simulink model "AUAV_V3_TestMavLink"  (Simulink 7.8)
settings: Solver=FixedStepDiscrete  StartTime=0.0  StopTime=10.0  FixedStep=T  RelTol=1e-3
PreLoadFcn:
  | T = 0.005;
  | MavlinkBus;
values from neighbouring files (symbols this model uses):
  mavlink_raw_imu_t = Simulink.Bus    [MavlinkBus.m]
undefined symbols (not defined in the file or in its folder): A0, A2, A3, A6, B0, D0, F2, F3, G15, P127, P16, P64, P82, P83, P98, P99, Pin, Timer
libraries: MCHP_Blockset x22, simulink x4
Description:
  | Rapid Prototyping model.
  | Require the MPLAB Blockset for Simulink v3.30 or above. [http://www.microchip.com/SimulinkBlocks]
  | Author: Lubin Kerhuel
  | 
  | Get AGM sensors raw values from the UAV V3 board from Asrovtech. [http://arsovtech.com/?p=1414]
settings Model: Creator=M91449  LastModifiedBy=UglyRed
settings OptimizationCC: InlineParams=on  InlineInvariantSignals=on  EnhancedBackFolding=on  ExpressionDepthLimit=128  OptimizeModelRefInitCode=on  LifeSpan=1
settings DebuggingCC: MultiTaskDSMMsg=none  StateNameClashWarn=none
settings HardwareCC: ProdBitPerInt=16  ProdBitPerPointer=16  ProdLargestAtomicInteger=Integer  ProdIntDivRoundTo=Zero  ProdEndianess=LittleEndian  ProdWordSize=16  ProdHWDeviceType=Generic->Custom
settings RTWCC: SystemTargetFile=MCHP_dsPIC_stf.tlc  GenCodeOnly=on  TemplateMakefile=MCHP_dsPIC.tmf  Description=Microchip Embedded Target PIC24 dsPIC30 dsPIC33 (real-time)  GenerateReport=on  ProcessScript=MCHP_dsPIC_stf_make_rtw_hook  CustomSource=clib\MavlinkComm.c  IncludeHyperlinkInReport=on  LaunchReport=on  GenerateTraceInfo=on  GenerateTraceReport=on  GenerateTraceReportSl=on  GenerateTraceReportSf=on  GenerateTraceReportEml=on
settings RTWCC: CustomInclude=|
  | mavlink\include\common\
  | clib\
settings CodeAppCC: IgnoreCustomStorageClasses=off  CustomSymbolStrType=$N$R$M_T
settings STFCustomTargetCC: TargetLibSuffix=_lib.a  IncludeMdlTerminateFcn=off  GeneratePreprocessorConditionals=Use local settings  CombineOutputUpdateFcns=on  SuppressErrorStatus=on  ERTCustomFileBanners=on  SupportContinuousTime=off  SystemTargetFile=MCHP_dsPIC_stf.tlc
settings ERTTargetCC: TargetLibSuffix=_lib.a  MultiwordLength=2048  ParMdlRefBuildCompliant=off  CompOptLevelCompliant=off  ConcurrentExecutionCompliant=off  IncludeMdlTerminateFcn=off  SuppressErrorStatus=on  ERTFirstTimeCompliant=off  SupportNonInlinedSFcns=on  ModelStepFunctionPrototypeControlCompliant=off  CPPClassGenCompliant=off  ExtModeMexFile=noextcomm  InlinedParameterPlacement=NonHierarchical  ERTSrcFileBannerTemplate=MCHP_dsPIC_code_template.cgt  ERTHdrFileBannerTemplate=MCHP_dsPIC_code_template.cgt  ERTDataSrcFileTemplate=MCHP_dsPIC_code_template.cgt  ERTDataHdrFileTemplate=MCHP_dsPIC_code_template.cgt  ERTCustomFileTemplate=MCHP_main.tlc  ConvertIfToSwitch=off  SuppressUnreachableDefaultCases=off
settings CustomProperty: DataType=string  Value=33EP512MU810
settings EnumStrPairs: String=elf

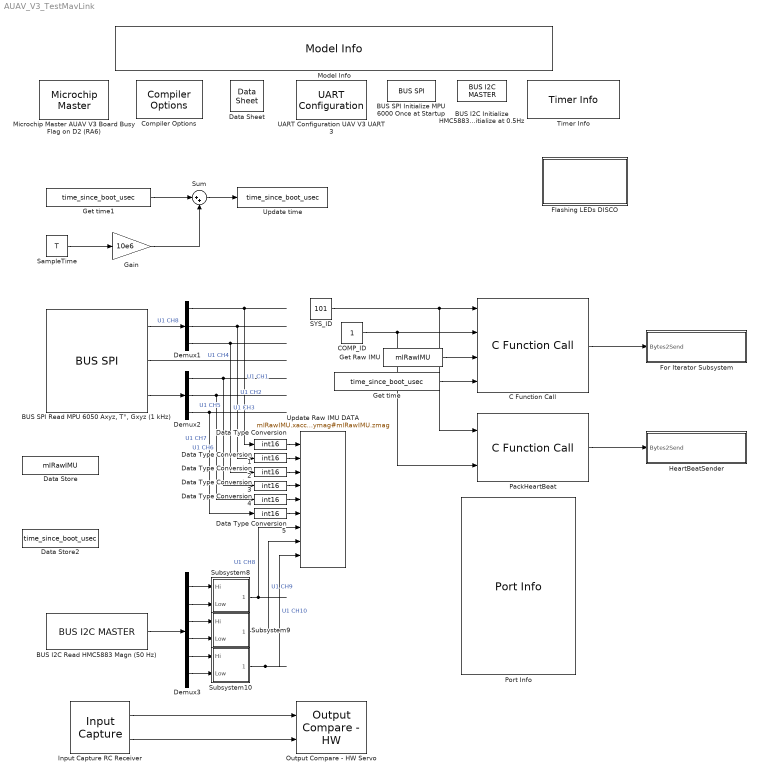
== system AUAV_V3_TestMavLink ==
  BUS I2C Initialize HMC5883 re-initialize at 0.5Hz : MCHP_Blockset/BUS I2C/BUS I2C MASTER  I2CRef=2  I2C_IntPriority=6  I2Csequence_txt="Initial-Configuration$     ---     $Start$Write Address:{[0x1E]}    % HMC5883L Address$Write Data (x1)  Write:{[0x00 0x78 0x00 0x00]}      % Configure$Stop"  I2Csequence_num=[BFF0000000000000 40E0600000000000 41186A0000000000 4118666E3C87173F]$[4070000000000000]$[3FF0000000000000 40E0200000000000 40F86A0000000000 40F866E066594CA2]$[4040000000000000 0000000000000000 0000000000000000 403E000000000000]$[4050000000000000 3FF0000000000000 0000000000000000 0000000000000000 405E000000000000 0000000000000000 0000000000000000]$[4000000000000000 40E0600000000000 40F86A0000000000 40F866E066594CA2]  InitialConfigurationNum=0  PIN_SDA_TXT=A3 / Pin[59]  PIN_SCL_TXT=A2 / Pin[58]  S_INPUT="[5  5]"  S_OUTPUT=[5]  S_INPUT_Size="[2  2]"  S_OUTPUT_Size=[4]  BlockingMode=off  SampleTime=.5  MCHP_MASTERLINK=|  MCHP_PORT={I2C 2 Clock}{SCL2}13:0:A2;{I2C 2 SDA}{SDA2}13:0:A3;  ORDERING=0
      | AUAV_V3_TestMavLink/Microchip Master
      | AUAV V3 Board
      | Busy Flag on D2 (RA6)
  BUS I2C Read HMC5883 Magn (50 Hz) : MCHP_Blockset/BUS I2C/BUS I2C MASTER  I2CRef=2  I2C_IntPriority=6  I2Csequence_txt="Initial-Configuration$     ---     $Start$Write Address:{[0x1E]}    % HMC5883L Address$Write Data (x1)  Write:{[0x3]}  $Stop$Start$Write Address:{[0x1E]}    % HMC5883L Address$Read Data (x6)  Read:{Out 5}$Stop"  I2Csequence_num=[BFF0000000000000 40E0600000000000 41186A0000000000 4118666E3C87173F]$[4070000000000000]$[3FF0000000000000 40E0200000000000 40F86A0000000000 40F866E066594CA2]$[4040000000000000 0000000000000000 0000000000000000 403E000000000000]$[4050000000000000 3FF0000000000000 0000000000000000 4008000000000000]$[4000000000000000 40E0600000000000 40F86A0000000000 40F866E066594CA2]$[3FF0000000000000 40E0200000000000 40F86A0000000000 40F866E066594CA2]$[4040000000000000 0000000000000000 0000000000000000 403E000000000000]$[4060000000000000 4018000000000000]$[4000000000000000 40E0600000000000 40F86A0000000000 40F866E066594CA2]  InitialConfigurationNum=0  PIN_SDA_TXT=A3 / Pin[59]  PIN_SCL_TXT=A2 / Pin[58]  S_INPUT="[5  5]"  S_OUTPUT=[5]  S_INPUT_Size="[2  2]"  S_OUTPUT_Size=[4]  BlockingMode=off  SampleTime=T  MCHP_MASTERLINK=|  MCHP_PORT={I2C 2 Clock}{SCL2}13:0:A2;{I2C 2 SDA}{SDA2}13:0:A3;  ORDERING=0
      | AUAV_V3_TestMavLink/Microchip Master
      | AUAV V3 Board
      | Busy Flag on D2 (RA6)
  BUS SPI Initialize MPU 6000 Once at Startup : MCHP_Blockset/BUS SPI/BUS SPI  SPIRef=1  DMA="[0  2  3]"  SPI_IntPriority=5  SPIsequence_txt="Initial-Configuration$     ---     $Set Port E4 / Pin[100] to 1    % /CS$Delay of 0.01(s)$Set Port E4 / Pin[100] to 0    % /CS$Write only (x1)  Write:{[0x6B80]}      % PWR_MGMT_1, BIT_H_RESET$Set Port E4 / Pin[100] to 1    % /CS$Delay of 0.06(s)$Set Port E4 / Pin[100] to 0    % /CS$Write only (x1)  Write:{[0x6B03]}      % PWR_MGMT_1, MPU_CLK_SEL_PLLGYROZ - PLL with Y axis gyroscope reference$Set Port E4 / Pin[100] to 1    % /CS$Delay of 0.01(s)$Set Port E4 / Pin[100] to 0    % /CS$Write only (x1)  Write:{[0x6A10]}      % conf Pow Mngt 1$Set Port E4 / Pin[100] to 1    % /CS$Set Port E4 / Pin[100] to 0    % /CS$Write only (x1)  Write:{[0x1904]}      % Sample rate = 200Hz  Fsample= 1Khz/(N+1) = 200Hz$Set Port E4 / Pin[100] to 1$Set Port E4 / Pin[100] to 0$Write only (x1)  Write:{[0x1A03]}      % LPF - Gyro 42Hz 4.8mS delay - Accel 44Hz 4.9mS delay$Set Port E4 / Pin[100] to 1$Set Port E4 / Pin[100] to 0$Write only (x1)  Write:{[0x1B08]}      % Gyro scale 500º/s$Set Port E4 / Pin[100] to 1$Set Port E4 / Pin[100] to 0$Write only (x1)  Write:{[0x3709]}      % INT_PIN_CFG, BIT_INT_LEVEL | BIT_INT_RD_CLEAR$Set Port E4 / Pin[100] to 1$Set Port E4 / Pin[100] to 0$Write only (x1)  Write:{[0x3801]}      % INT: Raw data ready$Set Port E4 / Pin[100] to 1"  SPIsequence_num=[BFF0000000000000 4091D00000000000 0000000000000000 40E0000000000000 4116409C00000000 4116409D55555555]$[4070000000000000]$[4010000000000000 4051000000000000 3FF0000000000000]$[4020000000000000 3F847AE147AE147B]$[4010000000000000 4051000000000000 0000000000000000]$[3FF0000000000000 3FF0000000000000 0000000000000000 40DAE00000000000]$[4010000000000000 4051000000000000 3FF0000000000000]$[4020000000000000 3FAEB851EB851EB8]$[4010000000000000 4051000000000000 0000000000000000]$[3FF0000000000000 3FF0000000000000 0000000000000000 40DAC0C000000000]$[4010000000000000 4051000000000000 3FF0000000000000]$[4020000000000000 3F847AE147AE147B]$[4010000000000000 4051000000000000 0000000000000000]$[3FF0000000000000 3FF0000000000000 0000000000000000 40DA840000000000]$[4010000000000000 4051000000000000 3FF0000000000000]$[4010000000000000 4051000000000000 0000000000000000]$[3FF0000000000000 3FF0000000000000 0000000000000000 40B9040000000000]$[4010000000000000 4051000000000000 3FF0000000000000]$[4010000000000000 4051000000000000 0000000000000000]$[3FF0000000000000 3FF0000000000000 0000000000000000 40BA030000000000]$[4010000000000000 4051000000000000 3FF0000000000000]$[4010000000000000 4051000000000000 0000000000000000]$[3FF0000000000000 3FF0000000000000 0000000000000000 40BB080000000000]$[4010000000000000 4051000000000000 3FF0000000000000]$[4010000000000000 4051000000000000 0000000000000000]$[3FF0000000000000 3FF0000000000000 0000000000000000 40CB848000000000]$[4010000000000000 4051000000000000 3FF0000000000000]$[4010000000000000 4051000000000000 0000000000000000]$[3FF0000000000000 3FF0000000000000 0000000000000000 40CC008000000000]$[4010000000000000 4051000000000000 3FF0000000000000]  PIN_SDI_TXT=E3 / P83 / Pin[99]  PIN_SDO_TXT=E2 / P82 / Pin[98]  PIN_SCK_TXT=G15 / P127 / Pin[1]  PIN_SS_TXT=B0 / Pin[21]  S_INPUT="[5  5]"  S_OUTPUT=[5]  S_INPUT_Size="[2  2]"  S_OUTPUT_Size=[4]  BlockingMode=off  SampleTime=inf  MCHP_MASTERLINK=|  MCHP_PORT={SPI 1 input}{SDI1}12:0:P83;{SPI 1 output}{SDO1}12:1:P82;{SPI 1 Clock output}{SCK1}12:1:P127;{SPI 1 Digital output}{SPI1-DOU}12:1:E4;{SPI 1 Digital output}{SPI1-DOU}12:1:E4;{SPI 1 Digital output}{SPI1-DOU}12:1:E4;{SPI 1 Digital output}{SPI1-DOU}12:1:E4;{SPI 1 Digital output}{SPI1-DOU}12:1:E4;{SPI 1 Digital output}{SPI1-DOU}12:1:E4;{SPI 1 Digital output}{SPI1-DOU}12:1:E4;{SPI 1 Digital output}{SPI1-DOU}12:1:E4;{SPI 1 Digital output}{SPI1-DOU}12:1:E4;{SPI 1 Digital output}{SPI1-DOU}12:1:E4;{SPI 1 Digital output}{SPI1-DOU}12:1:E4;{SPI 1 Digital output}{SPI1-DOU}12:1:E4;{SPI 1 Digital output}{SPI1-DOU}12:1:E4;{SPI 1 Digital output}{SPI1-DOU}12:1:E4;{SPI 1 Digital output}{SPI1-DOU}12:1:E4;{SPI 1 Digital output}{SPI1-DOU}12:1:E4;{SPI 1 Digital output}{SPI1-DOU}12:1:E4;  ORDERING=0
      | AUAV_V3_TestMavLink/Microchip Master
      | AUAV V3 Board
      | Busy Flag on D2 (RA6)
  "BUS SPI Read MPU 6050 Axyz, T°, Gxyz (1 kHz)" : MCHP_Blockset/BUS SPI/BUS SPI  SPIRef=1  DMA="[0  2  3]"  SPI_IntPriority=5  SPIsequence_txt="Initial-Configuration$     ---     $Set Port E4 / Pin[100] to 0    % /CS$Write only (x1)  Write:{[0xBA00]}      % read one byte before$Read only (x3)  Read:{Axyz}    % Accelerometers$Read only (x1)  Read:{T°}    % Temperature$Read only (x3)  Read:{Gxyz}    % rate gyros$Set Port E4 / Pin[100] to 1    % /CS"  SPIsequence_num=[BFF0000000000000 4091D00000000000 0000000000000000 40E0000000000000 4116409C00000000 4116409D55555555]$[4070000000000000]$[4010000000000000 4051000000000000 0000000000000000]$[3FF0000000000000 3FF0000000000000 0000000000000000 40E7400000000000]$[4000000000000000 4008000000000000]$[4000000000000000 3FF0000000000000]$[4000000000000000 4008000000000000]$[4010000000000000 4051000000000000 3FF0000000000000]  PIN_SDI_TXT=E3 / P83 / Pin[99]  PIN_SDO_TXT=E2 / P82 / Pin[98]  PIN_SCK_TXT=G15 / P127 / Pin[1]  PIN_SS_TXT=B0 / Pin[21]  S_INPUT="[5  5]"  S_OUTPUT=[5]  S_INPUT_Size="[2  2]"  S_OUTPUT_Size=[4]  BlockingMode=off  SampleTime=T  MCHP_MASTERLINK=|  MCHP_PORT={SPI 1 input}{SDI1}12:0:P83;{SPI 1 output}{SDO1}12:1:P82;{SPI 1 Clock output}{SCK1}12:1:P127;{SPI 1 Digital output}{SPI1-DOU}12:1:E4;{SPI 1 Digital output}{SPI1-DOU}12:1:E4;  ORDERING=0
      | AUAV_V3_TestMavLink/Microchip Master
      | AUAV V3 Board
      | Busy Flag on D2 (RA6)
  C Function Call : MCHP_Blockset/User Functions/C Function Call  ParseFilesChkbx=off  ListFunctions1=Custom Function  Function1=uint8_t PackRawIMU(uint8_t system_id, uint8_t component_id, mavlink_raw_imu_t mlRawIMUData ,uint32_t time_usec)  AddHeaderDeclaration=on  Function1Type=when block is updated (default)  Fct1BlockIn="system_id  , component_id  , mlRawIMUData  , time_usec"  FctReturnBlockOut=on  ORDERING=None  SampleTime=0.02  MCHP_MASTERLINK=|  PinDigitalInput=[]  PinDigitalOutput=[]  PinAnalogInput=[]
      | AUAV_V3_TestMavLink/Microchip Master
      | AUAV V3 Board
      | Busy Flag on D2 (RA6)
  COMP_ID : Constant  OutDataTypeStr=uint8
  Compiler Options : MCHP_Blockset/System Configuration/Compiler Options  Priority=1  LATEST_CMPLR=on  COMP_LIST=Dynamic Options  COMP_LIST_TXT=xc16 - v1.21  USE_64BIT_DOUBLE=off  MCHP_MULTITHREAD_COMPILATION=off  MCHP_MASTERLINK=|  OPTIMIZATION_LEVEL=3  MCONST=in code memory  MPLAB_LINKLIB=default  MPLAB_LINKLIB1=default  UNROLL_LOOPS=off  OMIT_FRAME_POINTER=off  PROCEDURAL_ABSTRACTION=off  HEAP_SIZE=0  OMF=elf  DEBUG_INFO=off  AssemblyListing=off  ProduceHexOutput=off
      | AUAV_V3_TestMavLink/Microchip Master
      | AUAV V3 Board
      | Busy Flag on D2 (RA6)
  Data Sheet : MCHP_Blockset/System Info/Data Sheet  DOC_MCHP_Id=33EP512MU810  DOC_FilePath=C:\Users\M91449\AppData\Local\Temp\70616g.pdf  DOC_FileLastCheckTime="[2013             11             10             22              4         17.021]"  cpy_MCHP_Id=33EP512MU810  MCHP_MASTERLINK=|
      | AUAV_V3_TestMavLink/Microchip Master
      | AUAV V3 Board
      | Busy Flag on D2 (RA6)
      settings: AttributesFormatString=%<cpy_MCHP_Id>
  Data Store : DataStoreMemory  DataStoreName=mlRawIMU  ReadBeforeWriteMsg=warning  WriteAfterWriteMsg=warning  WriteAfterReadMsg=warning  OutDataTypeStr=Bus:mavlink_raw_imu_t
  Data Store2 : DataStoreMemory  DataStoreName=time_since_boot_usec  ReadBeforeWriteMsg=warning  WriteAfterWriteMsg=warning  WriteAfterReadMsg=warning  OutDataTypeStr=uint32
  Data Type Conversion{,1..5} (6 alike) : DataTypeConversion  OutDataTypeStr=int16
  Demux1 : Demux  Outputs=3
  Demux2 : Demux  Outputs=3
  Demux3 : Demux  Outputs=6
  Flashing LEDs DISCO : Subsystem
  For Iterator Subsystem : Subsystem  TreatAsAtomicUnit=on
  Gain : Gain  Gain=10e6
  Get Raw IMU : DataStoreRead  DataStoreName=mlRawIMU  DataStoreElements=mlRawIMU
  Get time : DataStoreRead  DataStoreName=time_since_boot_usec  DataStoreElements=time_since_boot_usec
  Get time1 : DataStoreRead  DataStoreName=time_since_boot_usec  DataStoreElements=time_since_boot_usec
  HeartBeatSender : Subsystem  TreatAsAtomicUnit=on
  Input Capture RC Receiver : MCHP_Blockset/Pulse Input//Output/Input Capture  IntPriority=7  Channel="[1     2]"  Channel_OLD="[1  2]"  PIN_IC1=Dynamic Options  PIN_IC1_TXT=Dynamic Options  PIN_IC2=Dynamic Options  PIN_IC2_TXT=Dynamic Options  PIN_IC3=Dynamic Options  PIN_IC3_TXT=Dynamic Options  PIN_IC4=Dynamic Options  PIN_IC4_TXT=Dynamic Options  PIN_IC5=Dynamic Options  PIN_IC5_TXT=Dynamic Options  PIN_IC6=Dynamic Options  PIN_IC6_TXT=Dynamic Options  PIN_IC7=Dynamic Options  PIN_IC7_TXT=Dynamic Options  PIN_IC8=Dynamic Options  PIN_IC8_TXT=Dynamic Options  PIN_IC9=Dynamic Options  PIN_IC9_TXT=Dynamic Options  PIN_IC10=Dynamic Options  PIN_IC10_TXT=Dynamic Options  PIN_IC11=Dynamic Options  PIN_IC11_TXT=Dynamic Options  PIN_IC12=Dynamic Options  PIN_IC12_TXT=Dynamic Options  PIN_IC13=Dynamic Options  PIN_IC13_TXT=Dynamic Options  PIN_IC14=Dynamic Options  PIN_IC14_TXT=Dynamic Options  PIN_IC15=Dynamic Options  PIN_IC15_TXT=Dynamic Options  PIN_IC16=Dynamic Options  PIN_IC16_TXT=Dynamic Options  Channel_UP_Down_Periode="[1     1]"  MaxChannel="[0.003   0.003]"  SafeMarge="[0     0]"  MaxChannelValue="2.^[ 14.680  14.680]  =>  [26249  26249]"  ICxmax="[26249  26249]"  Timer="[1  1]"  ChangeDetected="[0     0]"  ChangeDetectedPortRef=3  SampleTime=-1  Status=OK  MCHP_TIMER_REQUEST="{Input Capture 1}{IC1}6:0:1:0:[1  2  3  4  5]:210000;{Input Capture 1}{IC1}6:0:1:0:[1  2  3  4  5]:210000;"  MCHP_TIMER_RESULT=[1 26249.000000000011 ;1 26249.000000000011 ]  MCHP_MASTERLINK=|
      | AUAV_V3_TestMavLink/Microchip Master
      | AUAV V3 Board
      | Busy Flag on D2 (RA6)
  Microchip Master AUAV V3 Board Busy Flag on D2 (RA6) : MCHP_Blockset/System Configuration/Microchip Master  Priority=1  PICREF=33EP512MU810  TIMESTEP_REF="Timer  ( 0.005s )"  BUSYFLAG=Dynamic Options  BUSYFLAG_TXT=A6 / Pin[91]  PWRTEN=PWRT enabled  BOREN=Disable  BODENV=2.7V  BORV=Brown-out Reset set at 2.0V  FPWRT=128ms  DSBOREN=Deep Sleep BOR enabled in Deep Sleep  DSLPBOR=Deep Sleep BOR enabled in Deep Sleep  MCLRE=Enabled  PMDL1WAY=Allow only one reconfiguration  RSTPRI=Device will obtain reset instruction from Primary flash  TEMP=Not used  SOSCSRC=Analog Mode for use with crystal  SOSCSEL=Secondary oscillator configured for high-power operation  IOL1WAY=Allow only one reconfiguration  ALTVREF=Voltage reference input; ADC =RA9/RA10 Comparator =RA9;RA10  DISUVREG=Regulator is disabled  DSSWEN=Deep Sleep is controlled by the register bit DSEN  LPCFG=Disabled - regardless of RETEN  RTCBAT=RTC operation is continued through VBAT  VBTBOR=VBAT BOR enabled  WUTSEL=Default regulator start-up time used  POWERSAVE=off  FNOSC=Primary oscillator (XT; HS; EC)  FPR=ECIO w/ PLL 16x  FOSFPR=HS3 w/PLL 16x  FOS=Internal Fast RC  FRANGE=High Range  OSCILLATOR_SELECT=Crystal / Ceramic resonator  OSCILLATOR_SELECT_spd=Crystal / Ceramic resonator  QUARTZ=8e6  QUARTZ_spd=8e6  ACTIV_PLL=on  ACTIV_PLL_spd=on  MIPS_DESIRED=70e6  MIPS_DESIRED_spd=70e6  FPLLMUL=24x Multiplier  FPLLIDIV=8x Divider  POSCFREQ=Primary oscillator/external clock input frequency greater than 8MHz  POSCMD=XT Crystal Oscillator Mode  POSCMOD=Primary Oscillator Disabled  MIPS=70 * 1e6  FPLLODIV=32x Divider  PLLKEN=Clock switch to PLL source will wait until the PLL lock signal is valid.  FCKSM=Both Clock Switching and Fail-safe Clock Monitor are enabled  FCKSMEN=Sw Disabled; Mon Disabled  IESO=Start up with FRC; then switch  DSWDTPS=1:2;147;483;648 (25.7 Days)  FWDTEN=Disable  FWDTWINSZ=Window Size is 25%  FWPSA=1:512  FWPSA0=1:128  FWPSB=1:16  WDT=Disable  WDTPOST=1:32768  WDTPRE=1:128  WDTPS=1:32768  WINDIS=Watchdog Timer in Non-Window mode  WWDTEN=Non-Window mode  DSWDTEN=DSWDT enabled  DSWDTOSC=DSWDT uses Low Power RC Oscillator (LPRC)  FPBDIV=Pb_Clk is Sys_Clk/8  FSOSCEN=Enable SOSC  LPRCSEL=High Power; High Accuracy Mode  OSCIOFCN=OSCO/CLKO/RC15 functions as CLKO (FOSC/2)  OSCIOFNC=OSC2 is general purpose digital I/O pin  LVRCFG=Low Voltage regulator is not available  PLL_96MHZ=Enabled  PLL96MHZ=96 MHz PLL Startup is enabled automatically on start-up  PLLDIV=PLL is disabled  WDTCLK=WDT uses LPRC  WDTCMX=WDT clock source is determined by the WDTCLK Configuration bits  WDTWIN=WDT Window is 25% of WDT period  APL=Aux Flash Code protect is disabled  APLK=Aux Flash Write Protection and Code Protection is Disabled  AWRP=Auxiliary program memory is not write-protected  BSS=No boot program Flash segment  BWP=Protection Disabled  BWRP=Boot Segment may be written  CP=Protection Disabled  EBS=No Boot EEPROM  ESS=No Segment Data EEPROM  GCP=Disable  GSS=General Segment Code protect is disabled  GSS0=No protection  GSSK=General Segment Write Protection and Code Protection is Disabled  GWRP=General Segment may be written  PWP=Disable  RBS=No Boot RAM  RSS=No Secure RAM  SSS=No Secure Segment  SWRP=Secure segment may be written  WPCFG=Disable  WPDIS=Disable  WPEND=Write Protect from WPFP to the last page of memory  WPFP=Page 127 (0x1FC00)  ICESEL=Communicate on PGEC1/PGED1  ICS=Communicate on PGEC3 and PGED3  JTAGEN=Disable  COE=Reset Into Operational Mode  RES=Not used  DEBUG=Debugger is Disabled  BACKBUG=Not used  BKBUG=Device resets into Operational mode  ALTI2C=I2C mapped to SDA1/SCL1 pins  ALTI2C1=SDA1/SCK1 pins are selected as the I/O pins for I2C1  ALTI2C2=ASDA2/ASCK2 pins are selected as the I/O pins for I2C2  ALTQIO=QEA1; QEB1; INDX1 are selected as inputs to QEI1  ALTSS1=SS1A is selected as the I/O pin for SPI1  CMPPOL0=Hysteresis is applied to falling edge  CMPPOL1=Hysteresis is applied to falling edge  FCANIO=Default CAN I/O  FETHIO=Default Ethernet I/O  FMIIEN=MII Enabled  FSRSSEL=SRS Priority 7  FUSBIDIO=Controlled by the USB Module  FVBUSONIO=Controlled by USB Module  HPOL=Active High  HYST0=45 mV Hysteresis  HYST1=45 mV Hysteresis  I2C1SEL=Use Default SCL1/SDA1 Pins For I2C1  LPOL=Active High  PWMPIN=Control with PORT/TRIS regs  RTCOSC=RTCC uses Secondary Oscillator (SOSC)  UPLLEN=USB PLL is enabled  UPLLIDIV=12x Divider  ATMOD8=Not used  ALTPMP=EPMP pins are in default location mode  I2C2SEL=I2C2 is multiplexed to SDA2/RA3 and SCL2/RA2  ALTADREF=AVREF+/AVREF- are mapped to RA9/RA10  ALTCVREF=CVREF+/CVREF- are mapped to RA9/RA10  PWMLOCK=PWM registers may be written without key sequence  MCHP_TIMER_REQUEST={Time Step}{TS}0:2:3:1:[]:350000;  MCHP_TIMER_RESULT=[1 43748.999999999949 ]  MCHP_PORT={Busy Flag}{Busy}0:1:A6;  MCHP_PLLRegisters="[5    243  16385     -1]"  MCHPVAR="MCHP.id = '33EP512MU810';MCHP.idN = [33  512  810];MCHP.idL = {'EP','MU',''};MCHP.Arch =3;MCHP.Rx = reshape([17   25   -1   72   93   87   90   -1   -1   -1   -1   38   24    6   76   94   88   89   -1   -1   -1   -1   58   23    7   77   98   52   57   -1   -1   -1   -1   59   22    8   78   99   51   56   -1   -1   -1   -1   60   21    9   81  100   49   -1   -1   -1   -1   -1   61   20   -1   82    3   50   -1   -1   -1   -1   -1   91   26   -1   83    4   -1   10   -1   -1   -1   -1   92   27   -1   84    5   -1   11   -1   -1   -1   -1   -1   32   -1   68   18   53   12   -1   -1   -1   -1   28   33   -1   69   19   -1   14   -1   -1   -1   -1   29   34   -1   70   -1   -1   -1   -1   -1   -1   -1   -1   35   -1   71   -1   -1   -1   -1   -1   -1   -1   -1   41   63   79   -1   40   96   -1   -1   -1   -1   -1   42   73   80   -1   39   97   -1   -1   -1   -1   66   43   74   47   -1   -1   95   -1   -1   -1   -1   67   44   64   48   -1   -1    1   -1   -1   -1   -1],11,16);MCHP.RP = [-1   -1   -1   -1   -1   -1   -1   -1   -1   -1   -1   -1   -1   -1   -1   -1   -1   -1   -1   -1   -1   -1   -1   -1   -1   -1   -1   -1   -1   -1   -1   -1   -1   -1   -1   -1   -1   -1   -1   -1   -1   -1   -1   -1   -1   -1   -1   -1   -1   -1   -1   -1   -1   -1   -1   -1   -1   -1   -1   -1   -1   -1   -1   -1   48   49   50   51   52   53   54   55   -1   -1   -1   -1   -1   -1   -1   63   64   -1   66   -1   68   69   -1   71   -1   -1   -1   -1   -1   -1   -1   -1   80   81   82   83   84   85   -1   -1   88   -1   -1   -1   92   93   -1   -1   96   97   -1   -1   -1   -1  102   -1  104   -1   -1   -1   -1  109  110  111];MCHP.RPI = [-1   -1   -1   -1   -1   -1   -1   -1   -1   -1   -1   -1   -1   -1   -1   -1    0    1    2    3    4    5    6    7   -1   -1   -1   -1   -1   -1   14   15   16   17   18   19   20   21   22   23   24   25   26   27   28   29   30   31   -1   33   34   35   36   -1   -1   -1   -1   -1   -1   -1   44   45   46   -1   -1   -1   -1   -1   -1   -1   -1   -1   56   57   58   59   60   61   62   -1   -1   65   -1   67   -1   -1   70   -1   72   73   -1   -1   -1   -1   -1   -1   -1   -1   -1   -1   -1   -1   -1   -1   -1   -1   -1   -1   -1   -1   -1   -1   -1   -1   -1   -1   -1   -1   -1  103   -1  105   -1   -1  108];MCHP.PPS.reg_RPINRx = [-1  1  1  1  1 -1  1  1  1  1  1  1  1  1  1  1  1  1  1  1  1  1 -1 -1  1  1  1  1  1  1  1  1  1  1  1  1  1  1  1  1  1  1  1 -1 -1 -1  1 -1 -1 -1 -1 -1  1  1  1  1  1  1  1  1  1 -1  1  1  1 -1  1  1  1  1  1  1  1  1 -1  1  1  1  1  1  1  1  1 -1  1  1  1];MCHP.RPINR_list = {'1','INT1','INT2','INT3','INT4','6','T2CK','T3CK','T4CK','T5CK','T6CK','T7CK','T8CK','T9CK','IC1','IC2','IC3','IC4','IC5','IC6','IC7','IC8','OCFA','OCFB','FLT1','FLT2','FLT3','FLT4','QEA1','QEB1','INDX1','HOME1','QEA2','QEB2','INDX2','HOME2','U1RX','U1CTS','U2RX','U2CTS','SDI1','SCK1','SS1','44','SDI2','SCK2','SS2','48','CSDIR','CSCK','COFSIN','52','C1RX','C2RX','U3RX','U2CTS','U4RX','U4CTS','SDI3','SCK3','SS3','62','SDI4','SCK4','SS4','66','IC9','IC10','IC11','IC12','IC13','IC14','IC15','IC16','OCFC','SYNCI1','SYNCI2','DTCMP1','DTCMP2','DTCMP3','DTCMP4','DTCMP5','DTCMP6','DTCMP7','FLT5','FLT6','FLT7','88'};MCHP.RPOR_list = {'1','U1TX','U1RTS','U2TX','U2RTS','SDO1','SCK1','SS1','SDO2','SCK2','SS2','CSDO','CSCK','COFS','C1TX','C2TX','OC1','OC2','OC3','OC4','OC5','OC6','OC7','OC8','C1OUT','C2OUT','C3OUT','U3TX','U3RTS','U4TX','U4RTS','SDO3','SCK3','SS3','SDO4','SCK4','SS4','OC9','OC10','OC11','OC12','OC13','OC14','OC15','OC16','SYNCO1','SYNCO2','QEI1CCMP','QEI2CCMP','REFCLK','C4OUT'};MCHP.PPS.map_RPnR_RPORx = [64   65   66   67   68   69   70   71   79   80   82   84   85   87   96   97   98   99  100  101   -1   -1  104  108  109  112  113  118  120  125  126  127];MCHP.fcy.periph = 70000000;MCHP.TimeStepFactor = [1];MCHP.fcy.MIPS = 70000000;MCHP.TimeStep_Timer = 1;MCHP.NTIMERS = 9;MCHP.PowerSave = [0];MCHP.DMA.Num = [15];MCHP.DMA.CNTmax = [16383];MCHP.QEI.QEICONx = [49023  49023     -1     -1     -1     -1];MCHP.QEI.QEItype = [2];MCHP.QEI.Port_QEI_INDX = [-1 -1];MCHP.QEI.Port_QEI_QEA = [-1 -1];MCHP.QEI.Port_QEI_QEB = [-1 -1];MCHP.QEI.Port_QEI_UPDN = [-1 -1];MCHP.ADC.ADCONx = [47103  59391  40959    263      0      0];MCHP.ADC.ADCHS_0 = [40863   1799];MCHP.ADC.ANtype = [3  1];MCHP.ADC.Flags = [1  0];MCHP.ADC.Buffer = [16  16];MCHP.ADC.port = [16  17  18  19  20  21  22  23  24  25  26  27  28  29  30  31  33  34  35  36  72  73   6   7  64  65  66  67  68  69  70  71  -1  -1  -1  -1  -1  -1  -1  -1  -1  -1  -1  -1  -1  -1  -1  -1  -1  -1  -1  -1  -1  -1  -1  -1  -1];MCHP.ADC.port_VrefP = [-1];MCHP.ADC.port_VrefM = [-1];MCHP.ADC.port_AVdd = [-1];MCHP.ADC.port_AVss = [-1];MCHP.PWM_HS.Flags = [6  2  1];MCHP.PWM.port_FLT = [-1 -1 -1 -1 -1 -1 -1 -1 -1 -1 -1 -1 -1 -1 -1 -1 -1 -1 -1 -1 -1 -1 -1 -1 -1 -1 -1 -1 -1 -1 -1 -1 -1];MCHP.PWM.PWMRef = -1;MCHP.PWM.Flag = 0;MCHP.PWM.Port_PWM_l = [64  66  68  70  33  35  -1  -1  -1;-1 -1 -1 -1 -1 -1 -1 -1 -1];MCHP.PWM.Port_PWM_h = [65  67  69  71  34  36  -1  -1  -1;-1 -1 -1 -1 -1 -1 -1 -1 -1];MCHP.IC.Port = [32767  32767  32767  32767  32767  32767  32767  32767  32767  32767  32767  32767  32767  32767  32767  32767];MCHP.IC.type = 1;MCHP.OC.Port = [32767  32767  32767  32767  32767  32767  32767  32767  32767  32767  32767  32767  32767  32767  32767  32767];MCHP.OC.type = 1;MCHP.CN.Port = [-1 -1 -1 -1 -1 -1 -1 -1 -1 -1 -1 -1 -1 -1 -1 -1 -1 -1 -1 -1 -1 -1 -1 -1 -1 -1 -1 -1 -1 -1 -1 -1 -1 -1 -1 -1 -1 -1 -1 -1 -1 -1 -1 -1 -1 -1 -1 -1 -1 -1 -1 -1 -1 -1 -1 -1 -1 -1 -1 -1 -1 -1 -1 -1 -1 -1 -1 -1 -1 -1 -1 -1 -1 -1 -1 -1 -1 -1 -1 -1 -1 -1 -1 -1 -1];MCHP.CN.PullUp = [50943  65535  61470  65535   1023  12607  62403      0      0      0      0];MCHP.CN.type = 1;MCHP.CN.Flag_PullDown = 1;MCHP.SPI.Refs = [1  2  3  4  0  0];MCHP.SPI.SPIxCON1 = 8191;MCHP.SPI.SPIxCON2 = 57347;MCHP.SPI.Port_SDI = [-1  103   -1   -1   -1   -1];MCHP.SPI.Port_SDO = [-1  104   -1   -1   -1   -1];MCHP.SPI.Port_SCK = [-1  102   -1   -1   -1   -1];MCHP.SPI.Port_SS = [-1 -1 -1 -1 -1 -1];MCHP.I2C.Refs = [1  2  0  0  0];MCHP.I2C.I2CxCON = 49151;MCHP.I2C.NewRegName = 1;MCHP.I2C.Port_SDA = [-1  84  -1  -1  -1];MCHP.I2C.Port_SCL = [-1  85  -1  -1  -1];MCHP.I2C.Port_ASDA = [57   3  -1  -1  -1];MCHP.I2C.Port_ASCL = [58   2  -1  -1  -1];MCHP.I2C.Fuse_Port_SCL_SDA = [17  18  -1  -1  -1;1  1 -1 -1 -1];MCHP.I2C.Fuse_Port_ASCL_ASDA = [17  18  -1  -1  -1;2  2 -1 -1 -1];MCHP.Comp.Port_CVrefin = [-1];MCHP.Comp.Port_CVref = [26];MCHP.Comp.Port_CVref1O = [-1];MCHP.Comp.Port_CVref2O = [-1];MCHP.Comp.Port_CxOUT = [32767  32767  32767     -1     -1];MCHP.Comp.Port_OAxOUT = [-1 -1 -1 -1 -1];MCHP.Comp.Port_CxINP = [21  19  55  -1  -1];MCHP.Comp.Port_CxINM = [103   20  102   -1;105   18  104   -1;46  54  45  -1;-1 -1 -1 -1;-1 -1 -1 -1];MCHP.Comp.nComp = [3  0  0];MCHP.Comp.OpAmp = [0];MCHP.Comp.CVRCON = [2047     0];MCHP.UART.port_Rx = [32767  32767  32767  32767     -1     -1];MCHP.UART.port_Tx = [32767  32767  32767  32767     -1     -1];MCHP.UART.port_ARx = [-1 -1];MCHP.UART.port_ATx = [-1 -1];MCHP.UART.port_RTS = [32767  32767  32767  32767     -1     -1];MCHP.UART.port_CTS = [32767  32767  32767  32767     -1     -1];MCHP.UART.reg_UxMODE = [48127  48127  48127  48127     -1     -1];MCHP.UART.reg_UxSTA = [61439  61439  61439  61439     -1     -1];"  MCHP_CRC=-1128758  BTMODE=Device is in Single Boot (legacy) mode  RES1=Not used  PLLSS=PLL is fed by the Primary oscillator  RES2=Not used  ALTCMPI=C1INC is on RB13; C2INC is on RB9 and C3INC is on RA0  BOREN1=BOR Enabled [When BOREN=1]  ALTRB6=Append the RP6/ASCL1/PMPD6 functions of RB6 to RA1 pin functions  RETCFG=Retention regulator is not available  DFMCY=48 Tcy  BSS2=No Boot Segment  CWRP=Configuration Segment may be written  CSS=No Protection (other than CWRP)  AIVTDIS=Disabled AIVT  BSLIM=Not used  WDTEN=Disable  BTSWP=Not used  DBCC=Not used  CTXT1=Not Assigned  CTXT2=Not Assigned  SEQNUM=Not used  nSEQNUM=Not used  BOREN0=Enabled  DMTIVT=Not used  DMTCNT=2^31 (2147483648)  DMTEN=Dead Man Timer is Enabled and cannot be disabled by software  ON=Not used  USERID=Not used  RESERVED1=Not used  PGL1WAY=Allow only one reconfiguration  FPLLRNG=34-68 MHz Input  FPLLICLK=FRC is input to the System PLL  FPLLMULT=PLL Multiply by 128  UPLLFSEL=USB PLL input is 24 MHz  DMTINTV=Window/Interval value is 127/128 counter value  WDTSPGM=WDT stops during Flash programming  FDMTEN=Deadman Timer is disabled  TRCEN=Trace features in the CPU are enabled  BOOTISA=Boot code and Exception code is MIPS32  FECCCON=ECC and Dynamic ECC are disabled (ECCCON bits are writable)  FSLEEP=Flash is powered down when the device is in Sleep mode  DBGPER=Allow CPU access to all permission regions  EJTAGBEN=Normal EJTAG functionality  TSEQ=Not used  CSEQ=Not used
  Model Info : simulink/Model-Wide Utilities/Model Info  InitialBlockCM=none  BlockCM=None  Frame=off  DisplayStringWithTags=%<Description>  HorizontalTextAlignment=Center  LeftAlignmentValue=0.5  SourceBlockDiagram=AUAV_V3_TestMavLink  TagMaxNumber=20
  Output Compare - HW Servo : MCHP_Blockset/Pulse Input//Output/Output Compare - HW  Channel="[1     2]"  Channel_OLD="[1     2]"  PIN_OC1=Dynamic Options  PIN_OC1_TXT=D0 / P64 / Pin[72]  PIN_OC2=Dynamic Options  PIN_OC2_TXT=D0 / P64 / Pin[72]  PIN_OC3=Dynamic Options  PIN_OC3_TXT=D0 / P64 / Pin[72]  PIN_OC4=Dynamic Options  PIN_OC4_TXT=D0 / P64 / Pin[72]  PIN_OC5=Dynamic Options  PIN_OC5_TXT=D0 / P64 / Pin[72]  PIN_OC6=Dynamic Options  PIN_OC6_TXT=D0 / P64 / Pin[72]  PIN_OC7=Dynamic Options  PIN_OC7_TXT=D0 / P64 / Pin[72]  PIN_OC8=Dynamic Options  PIN_OC8_TXT=D0 / P64 / Pin[72]  PIN_OC9=Dynamic Options  PIN_OC9_TXT=D0 / P64 / Pin[72]  PIN_OC10=Dynamic Options  PIN_OC10_TXT=D0 / P64 / Pin[72]  PIN_OC11=Dynamic Options  PIN_OC11_TXT=D0 / P64 / Pin[72]  PIN_OC12=Dynamic Options  PIN_OC12_TXT=D0 / P64 / Pin[72]  PIN_OC13=Dynamic Options  PIN_OC13_TXT=D0 / P64 / Pin[72]  PIN_OC14=Dynamic Options  PIN_OC14_TXT=D0 / P64 / Pin[72]  PIN_OC15=Dynamic Options  PIN_OC15_TXT=D0 / P64 / Pin[72]  PIN_OC16=Dynamic Options  PIN_OC16_TXT=D0 / P64 / Pin[72]  PIN_OCFA=Dynamic Options  PIN_OCFA_TXT=A0 / P16 / Pin[17]  PIN_OCFB=Dynamic Options  PIN_OCFB_TXT=A0 / P16 / Pin[17]  PIN_OCFC=Dynamic Options  PIN_OCFC_TXT=A0 / P16 / Pin[17]  Channel_UP_Down_Periode="[5     5]"  PulseTrig=Single pulse triggered by block execution  InputPeriod=are set to the Max time (constant below)  MaxChannel="[0.003   0.003]"  MaxChannelUnique=.0001  MaxChannelValue="2.^[ 14.680  14.680]  =>  [26249  26249]"  OCxmax="[26249  26249]"  Timer="[1  1]"  SampleTime=.02  MCHP_PORT={Output Compare 1}{OC1}7:1:P64;{Output Compare 2}{OC2}7:1:P64;  MCHP_TIMER_REQUEST="{Output Compare 1}{OC1}7:0:1:0:[1  2  3  4  5]:210000;{Output Compare 1}{OC1}7:0:1:0:[1  2  3  4  5]:210000;"  MCHP_TIMER_RESULT=[1 26249.000000000011 ;1 26249.000000000011 ]  MCHP_MASTERLINK=|
      | AUAV_V3_TestMavLink/Microchip Master
      | AUAV V3 Board
      | Busy Flag on D2 (RA6)
  PackHeartBeat : MCHP_Blockset/User Functions/C Function Call  ParseFilesChkbx=on  ListFunctions1=Custom Function  Function1=uint16_t PackHeartBeat(uint8_t system_id, uint8_t component_id)  AddHeaderDeclaration=on  Function1Type=when block is updated (default)  Fct1BlockIn="system_id  , component_id"  FctReturnBlockOut=on  DataCollected="s.chksm={ '563309-Jan-2015 23:25:22'};s.File1=reshape({ '  uint16_t  PackHeartBeat(uint8_t system_id, uint8_t component_id)','  uint16_t  PackRawIMU(uint8_t system_id, uint8_t component_id, mavlink_raw_imu_t mlRawIMUData ,uint32_t time_usec)','  char  sendQGCDebugMessage(const char * dbgMessage, char severity, unsigned char* bytesToAdd, char positionStart)','  uint8_t  GetCharAtBuffIdx(int32_t idx)'},1,4);"  ORDERING=None  SampleTime=0.5  MCHP_MASTERLINK=|  PinDigitalInput=[]  PinDigitalOutput=[]  PinAnalogInput=[]
      | AUAV_V3_TestMavLink/Microchip Master
      | AUAV V3 Board
      | Busy Flag on D2 (RA6)
  Port Info : MCHP_Blockset/System Info/Port Info  MCHP_MASTERLINK=|
      | AUAV_V3_TestMavLink/Microchip Master
      | AUAV V3 Board
      | Busy Flag on D2 (RA6)
  SYS_ID : Constant  Value=101  OutDataTypeStr=uint8
  SampleTime : Constant  Value=T  OutDataTypeStr=uint8
  Subsystem10 : Subsystem
  Subsystem8 : Subsystem
  Subsystem9 : Subsystem
  Sum : Sum  Inputs=|++
  Timer Info : MCHP_Blockset/System Info/Timer Info  MCHP_MASTERLINK=|
      | AUAV_V3_TestMavLink/Microchip Master
      | AUAV V3 Board
      | Busy Flag on D2 (RA6)
  UART Configuration UAV V3 UART 3 : MCHP_Blockset/BUS UART/UART Configuration  UART_REF=1  BAUD_Choice=Dynamic Options  BAUD_Choice_TXT="115200         [-0.06%]"  BAUD_Choice_IR=Dynamic Options  BAUD_Choice_IR_TXT=[]  BAUD_Custom=115200  IRDA=off  ALT_IO=on  PIN_RX=Dynamic Options  PIN_RX_TXT=F2 / P98 / Pin[52]  PIN_TX=Dynamic Options  PIN_TX_TXT=F3 / P99 / Pin[51]  FlowControl=None  PIN_CTS=Dynamic Options  PIN_CTS_TXT=A0 / P16 / Pin[17]  PIN_RTS=Dynamic Options  PIN_RTS_TXT=D0 / P64 / Pin[72]  MCHP_PORT="{UART1  Tx}{U1TX}3:1:P99;"  TX_IMPLEMENTATION=Circular Buffer  TX_INT_PRIORITY=1  TX_INT_WHEN=is empty & last char is sent  TX_CIRCULAR_SIZE=128  TX_DMA_CHANNEL="0   (Lowest Priority)"  TX_DMA_SIZE=[]  RX_IMPLEMENTATION=Do not implement Rx  RX_INT_PRIORITY=1  RX_INT_WHEN=receive 1 character  RX_CIRCULAR_SIZE=32  InitSequence_chkbox=on  BAUD_Choice_InitSeq=Dynamic Options  BAUD_Choice_InitSeq_TXT="110         [-0.00%]"  BAUD_Choice_IR_InitSeq=Dynamic Options  BAUD_Choice_IR_InitSeq_TXT=0  BAUD_Custom_InitSeq=0  InitSequence='Hello World'  MCHP_MASTERLINK=|
      | AUAV_V3_TestMavLink/Microchip Master
      | AUAV V3 Board
      | Busy Flag on D2 (RA6)
  Update Raw IMU DATA : DataStoreWrite  DataStoreName=mlRawIMU  DataStoreElements=mlRawIMU.xacc#mlRawIMU.yacc#mlRawIMU.zacc#mlRawIMU.xgyro#mlRawIMU.ygyro#mlRawIMU.zgyro#mlRawIMU.xmag#mlRawIMU.ymag#mlRawIMU.zmag
  Update time : DataStoreWrite  DataStoreName=time_since_boot_usec  DataStoreElements=time_since_boot_usec
  wires:
  "BUS SPI Read MPU 6050 Axyz, T°, Gxyz (1 kHz)"/1 -> Demux1/1  "U1 CH8"
  "BUS SPI Read MPU 6050 Axyz, T°, Gxyz (1 kHz)"/3 -> Demux2/1
  Demux1/3 -> Data Type Conversion2/1  "U1 CH3"
  Demux1/1 -> Data Type Conversion/1  "U1 CH1"
  Demux1/2 -> Data Type Conversion1/1  "U1 CH2"
  Demux2/1 -> Data Type Conversion3/1  "U1 CH5"
  Demux2/2 -> Data Type Conversion4/1  "U1 CH6"
  Demux2/3 -> Data Type Conversion5/1  "U1 CH7"
  "BUS SPI Read MPU 6050 Axyz, T°, Gxyz (1 kHz)"/2 -> ?  "U1 CH4"
  BUS I2C Read HMC5883 Magn (50 Hz)/1 -> Demux3/1
  Demux3/1 -> Subsystem8/1(Hi)
  Demux3/2 -> Subsystem8/2(Low)
  Demux3/3 -> Subsystem9/1(Hi)
  Demux3/4 -> Subsystem9/2(Low)
  Demux3/6 -> Subsystem10/2(Low)
  Demux3/5 -> Subsystem10/1(Hi)
  Subsystem9/1(Out1) -> Update Raw IMU DATA/8  "U1 CH9"
  Subsystem8/1(Out1) -> Update Raw IMU DATA/7  "U1 CH8"
  Subsystem10/1(Out1) -> Update Raw IMU DATA/9  "U1 CH10"
  Input Capture RC Receiver/2 -> Output Compare - HW Servo/2
  Input Capture RC Receiver/1 -> Output Compare - HW Servo/1
  SampleTime/1 -> Gain/1
  Get time1/1 -> Sum/1
  Gain/1 -> Sum/2
  Sum/1 -> Update time/1
  SYS_ID/1 -> C Function Call/1, PackHeartBeat/1
  COMP_ID/1 -> C Function Call/2, PackHeartBeat/2
  Get Raw IMU/1 -> C Function Call/3
  Get time/1 -> C Function Call/4
  Data Type Conversion/1 -> Update Raw IMU DATA/1
  Data Type Conversion1/1 -> Update Raw IMU DATA/2
  Data Type Conversion2/1 -> Update Raw IMU DATA/3
  Data Type Conversion3/1 -> Update Raw IMU DATA/4
  Data Type Conversion4/1 -> Update Raw IMU DATA/5
  Data Type Conversion5/1 -> Update Raw IMU DATA/6
  C Function Call/1 -> For Iterator Subsystem/1(Bytes2Send)
  PackHeartBeat/1 -> HeartBeatSender/1(Bytes2Send)

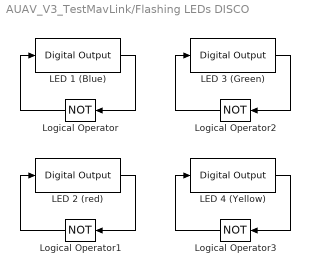
== system AUAV_V3_TestMavLink/Flashing LEDs DISCO ==
  LED 1 (Blue) : MCHP_Blockset/Digital IO/Digital Output  PORT=Dynamic Options  PORT_TXT="B   [ 0 : 15 ]"  PIN=2  PACK=off  SIMULTANEOUS=off  READPREVIOUS=on  ORDERING=None  SampleTime=.05  MCHP_MASTERLINK=|
      | AUAV_V3_TestMavLink/Microchip Master
      | AUAV V3 Board
      | Busy Flag on D2 (RA6)
  LED 2 (red) : MCHP_Blockset/Digital IO/Digital Output  PORT=Dynamic Options  PORT_TXT="B   [ 0 : 15 ]"  PIN=3  PACK=off  SIMULTANEOUS=off  READPREVIOUS=on  ORDERING=None  SampleTime=.1  MCHP_MASTERLINK=|
      | AUAV_V3_TestMavLink/Microchip Master
      | AUAV V3 Board
      | Busy Flag on D2 (RA6)
  LED 3 (Green) : MCHP_Blockset/Digital IO/Digital Output  PORT=Dynamic Options  PORT_TXT="B   [ 0 : 15 ]"  PIN=4  PACK=off  SIMULTANEOUS=off  READPREVIOUS=on  ORDERING=None  SampleTime=.25  MCHP_MASTERLINK=|
      | AUAV_V3_TestMavLink/Microchip Master
      | AUAV V3 Board
      | Busy Flag on D2 (RA6)
  LED 4 (Yellow) : MCHP_Blockset/Digital IO/Digital Output  PORT=Dynamic Options  PORT_TXT="B   [ 0 : 15 ]"  PIN=5  PACK=off  SIMULTANEOUS=off  READPREVIOUS=on  ORDERING=None  SampleTime=0.5  MCHP_MASTERLINK=|
      | AUAV_V3_TestMavLink/Microchip Master
      | AUAV V3 Board
      | Busy Flag on D2 (RA6)
  Logical Operator{,1..3} (4 alike) : Logic  Operator=NOT  AllPortsSameDT=off  OutDataTypeStr=boolean
  wires:
  LED 1 (Blue)/1 -> Logical Operator/1
  Logical Operator/1 -> LED 1 (Blue)/1
  LED 2 (red)/1 -> Logical Operator1/1
  Logical Operator1/1 -> LED 2 (red)/1
  LED 3 (Green)/1 -> Logical Operator2/1
  Logical Operator2/1 -> LED 3 (Green)/1
  LED 4 (Yellow)/1 -> Logical Operator3/1
  Logical Operator3/1 -> LED 4 (Yellow)/1

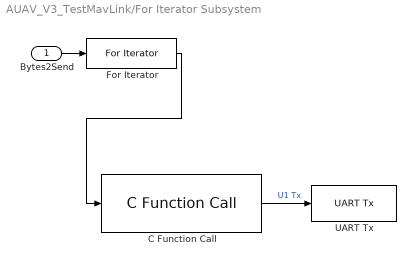
== system AUAV_V3_TestMavLink/For Iterator Subsystem ==
  Bytes2Send : Inport
  C Function Call : MCHP_Blockset/User Functions/C Function Call  ParseFilesChkbx=on  ListFunctions1=Custom Function  Function1=uint8_t GetCharAtBuffIdx(int32_t idx)  AddHeaderDeclaration=on  Function1Type=when block is updated (default)  Fct1BlockIn=idx  FctReturnBlockOut=on  DataCollected="s.chksm={ '514109-Jan-2015 22:49:09'};s.File1=reshape({ '  uint16_t  PackHeartBeat(void)','  uint16_t  PackRawIMU(uint8_t system_id, uint8_t component_id, mavlink_raw_imu_t mlRawIMUData ,uint32_t time_usec)','  char  sendQGCDebugMessage(const char * dbgMessage, char severity, unsigned char* bytesToAdd, char positionStart)','  uint8_t  GetCharAtBuffIdx(int32_t idx)'},1,4);"  ORDERING=None  SampleTime=-1  MCHP_MASTERLINK=|  PinDigitalInput=[]  PinDigitalOutput=[]  PinAnalogInput=[]
      | AUAV_V3_TestMavLink/Microchip Master
      | AUAV V3 Board
      | Busy Flag on D2 (RA6)
  For Iterator : ForIterator  IterationSource=external  IndexMode=Zero-based
  UART Tx : MCHP_Blockset/BUS UART/UART Tx  UART_REF=1  UART_String=off  ORDERING=None  SampleTime=-1  MCHP_MASTERLINK=|
      | AUAV_V3_TestMavLink/Microchip Master
      | AUAV V3 Board
      | Busy Flag on D2 (RA6)
  wires:
  Bytes2Send/1 -> For Iterator/1
  C Function Call/1 -> UART Tx/1  "U1 Tx"
  For Iterator/1 -> C Function Call/1

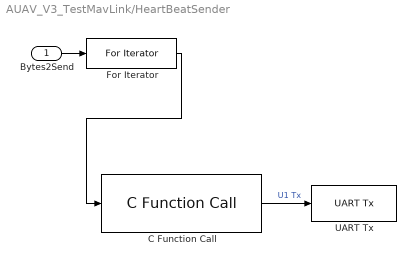
== system AUAV_V3_TestMavLink/HeartBeatSender ==
  Bytes2Send : Inport
  C Function Call : MCHP_Blockset/User Functions/C Function Call  ParseFilesChkbx=on  ListFunctions1=Custom Function  Function1=uint8_t GetCharAtBuffIdx(int32_t idx)  AddHeaderDeclaration=on  Function1Type=when block is updated (default)  Fct1BlockIn=idx  FctReturnBlockOut=on  DataCollected="s.chksm={ '514109-Jan-2015 22:49:09'};s.File1=reshape({ '  uint16_t  PackHeartBeat(void)','  uint16_t  PackRawIMU(uint8_t system_id, uint8_t component_id, mavlink_raw_imu_t mlRawIMUData ,uint32_t time_usec)','  char  sendQGCDebugMessage(const char * dbgMessage, char severity, unsigned char* bytesToAdd, char positionStart)','  uint8_t  GetCharAtBuffIdx(int32_t idx)'},1,4);"  ORDERING=None  SampleTime=-1  MCHP_MASTERLINK=|  PinDigitalInput=[]  PinDigitalOutput=[]  PinAnalogInput=[]
      | AUAV_V3_TestMavLink/Microchip Master
      | AUAV V3 Board
      | Busy Flag on D2 (RA6)
  For Iterator : ForIterator  IterationSource=external  IndexMode=Zero-based
  UART Tx : MCHP_Blockset/BUS UART/UART Tx  UART_REF=1  UART_String=off  ORDERING=None  SampleTime=-1  MCHP_MASTERLINK=|
      | AUAV_V3_TestMavLink/Microchip Master
      | AUAV V3 Board
      | Busy Flag on D2 (RA6)
  wires:
  For Iterator/1 -> C Function Call/1
  C Function Call/1 -> UART Tx/1  "U1 Tx"
  Bytes2Send/1 -> For Iterator/1

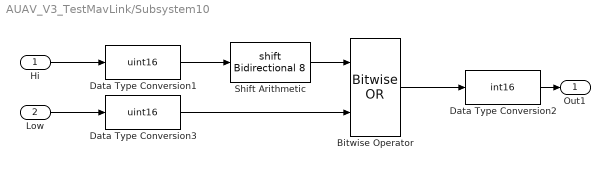
== system AUAV_V3_TestMavLink/Subsystem10 ==
  Hi : Inport
  Low : Inport  Port=2
  Bitwise Operator : simulink/Logic and Bit Operations/Bitwise Operator  logicop=OR  UseBitMask=off  NumInputPorts=2  BitMask=bin2dec('11011001')  BitMaskRealWorld=Stored Integer
  Data Type Conversion1 : DataTypeConversion  OutDataTypeStr=uint16  ConvertRealWorld=Stored Integer (SI)
  Data Type Conversion2 : DataTypeConversion  OutDataTypeStr=int16  ConvertRealWorld=Stored Integer (SI)
  Data Type Conversion3 : DataTypeConversion  OutDataTypeStr=uint16  ConvertRealWorld=Stored Integer (SI)
  Shift Arithmetic : ArithShift  BitShiftNumber=8
  Out1 : Outport
  wires:
  Hi/1 -> Data Type Conversion1/1
  Bitwise Operator/1 -> Data Type Conversion2/1
  Data Type Conversion2/1 -> Out1/1
  Data Type Conversion1/1 -> Shift Arithmetic/1
  Shift Arithmetic/1 -> Bitwise Operator/1
  Low/1 -> Data Type Conversion3/1
  Data Type Conversion3/1 -> Bitwise Operator/2

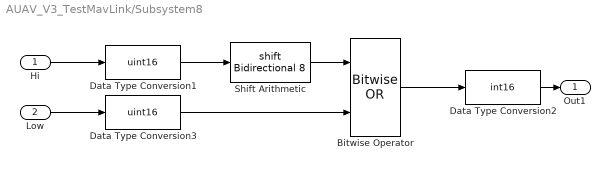
== system AUAV_V3_TestMavLink/Subsystem8 ==
  Hi : Inport
  Low : Inport  Port=2
  Bitwise Operator : simulink/Logic and Bit Operations/Bitwise Operator  logicop=OR  UseBitMask=off  NumInputPorts=2  BitMask=bin2dec('11011001')  BitMaskRealWorld=Stored Integer
  Data Type Conversion1 : DataTypeConversion  OutDataTypeStr=uint16  ConvertRealWorld=Stored Integer (SI)
  Data Type Conversion2 : DataTypeConversion  OutDataTypeStr=int16  ConvertRealWorld=Stored Integer (SI)
  Data Type Conversion3 : DataTypeConversion  OutDataTypeStr=uint16  ConvertRealWorld=Stored Integer (SI)
  Shift Arithmetic : ArithShift  BitShiftNumber=8
  Out1 : Outport
  wires:
  Hi/1 -> Data Type Conversion1/1
  Bitwise Operator/1 -> Data Type Conversion2/1
  Data Type Conversion2/1 -> Out1/1
  Data Type Conversion1/1 -> Shift Arithmetic/1
  Shift Arithmetic/1 -> Bitwise Operator/1
  Low/1 -> Data Type Conversion3/1
  Data Type Conversion3/1 -> Bitwise Operator/2

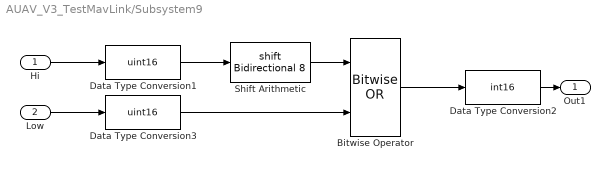
== system AUAV_V3_TestMavLink/Subsystem9 ==
  Hi : Inport
  Low : Inport  Port=2
  Bitwise Operator : simulink/Logic and Bit Operations/Bitwise Operator  logicop=OR  UseBitMask=off  NumInputPorts=2  BitMask=bin2dec('11011001')  BitMaskRealWorld=Stored Integer
  Data Type Conversion1 : DataTypeConversion  OutDataTypeStr=uint16  ConvertRealWorld=Stored Integer (SI)
  Data Type Conversion2 : DataTypeConversion  OutDataTypeStr=int16  ConvertRealWorld=Stored Integer (SI)
  Data Type Conversion3 : DataTypeConversion  OutDataTypeStr=uint16  ConvertRealWorld=Stored Integer (SI)
  Shift Arithmetic : ArithShift  BitShiftNumber=8
  Out1 : Outport
  wires:
  Data Type Conversion3/1 -> Bitwise Operator/2
  Low/1 -> Data Type Conversion3/1
  Shift Arithmetic/1 -> Bitwise Operator/1
  Data Type Conversion1/1 -> Shift Arithmetic/1
  Data Type Conversion2/1 -> Out1/1
  Bitwise Operator/1 -> Data Type Conversion2/1
  Hi/1 -> Data Type Conversion1/1
